simulink model "Matrix1"  (Simulink 9.0)
settings: Solver=FixedStepDiscrete  StartTime=0.0  StopTime=19800  FixedStep=200  RelTol=1e-3  EnableMultiTasking=on
settings Model: SuppressorTable=22 serialization::archive 11 0 6 0 0 0 0 0  Creator=scaife  LastModifiedBy=hbourbou  ExtModeAutoUpdateStatusClock=off
settings DataIOCC: ExternalInput=input_dataset  LimitDataPoints=on  SaveFormat=Dataset  SignalLoggingSaveFormat=ModelDataLogs  SaveState=on  SignalLoggingName=sigsOut
settings DebuggingCC: AlgebraicLoopMsg=error  SaveWithParameterizedLinksMsg=none  SignalResolutionControl=TryResolveAllWithWarning  MultiTaskDSMMsg=warning  MultiTaskCondExecSysMsg=none  StrictBusMsg=None
settings HardwareCC: TargetUnknown=on
settings SFSimCC: SimParseCustomCode=off
settings GRTTargetCC: GeneratePreprocessorConditionals=Disable all  CombineOutputUpdateFcns=off  GRTInterface=on  ExtMode=on

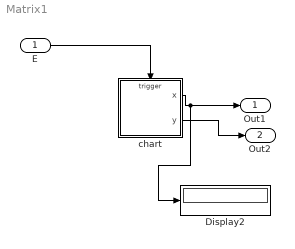
== system Matrix1 ==
  E : Inport
  Display2 : Display
  chart : Stateflow chart  TreatAsAtomicUnit=on
  Out1 : Outport
  Out2 : Outport  Port=2
  wires:
  E/1 -> chart/Trigger
  chart/1(x) -> Out1/1, Display2/1
  chart/2(y) -> Out2/1

== stateflow chart chart ==
  state A/
    en:
    i = 3;
    x(1) = x(2,i) + 1;
  state B/
    en:x(2) = x(2,2) + 1;
    y(2) = x(2) * 3;
  state C/
    en:x= y * 2;
  (default) -> A
  A -> B : E
  C -> A : E
  B -> C : E
  data: x output double size=[2 3] [0..100] =[1 2 3; 4 5 6]; i local int32; y output double size=[2 3] [0..100] =[1 2 3; 4 5 6]
  events: E input RISING_EDGE_EVENT
